simulink model "Prototype"  (R2015a)
settings: Solver=ode45  StartTime=0.0  StopTime=10.0  RelTol=1e-3
undefined symbols (not defined in the file): gray, jet, Rec, SDTV, strel
libraries: visionmorphops x2, visionsinks x2, visionconversions x1, visionanalysis x1, dspvision x1, visiontransforms x1
settings Model: Creator=Andrew H  LastModifiedBy=Andrew H

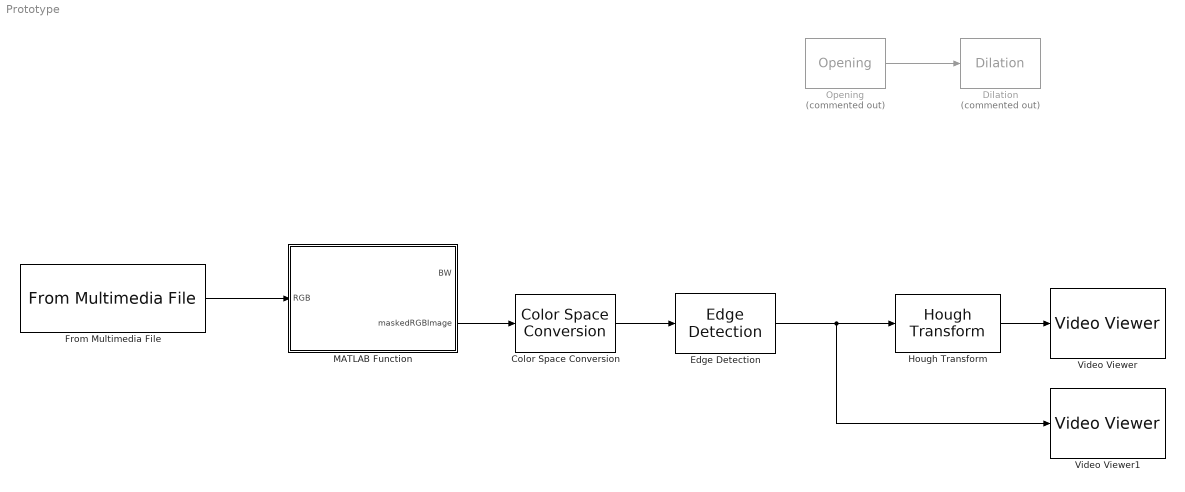
== system Prototype ==
  Color Space Conversion : visionconversions/Color Space  Conversion  conversion=Obsolete  conversionActive=R'G'B' to intensity  wp_str=D65  rec=Rec. 601 (SDTV)  sys=1125/60/2:1  imagePorts=One multidimensional signal
  Dilation : visionmorphops/Dilation  Commented=on  nhoodsrc=Specify via dialog  strel=[1 1; 1 1]
  Edge Detection : visionanalysis/Edge Detection  method=Sobel  outputType=Binary image  userDefinedThreshold=off  thresholdSource=Input port  threshold=20  thresholdTuning=4  edgeThinning=off  threshold_canny=[0.25 0.60]  autoPercent=70  sigma=1  prodOutputMode=Binary point scaling  prodOutputWordLength=32  prodOutputFracLength=8  roundingMode=Floor  overflowMode=off
  From Multimedia File : dspvision/From Multimedia File  inputFilename=C:\Users\Andrew H\Desktop\Video.mp4  loop=on  numPlays=inf  outputStreams=Video only  videoDataType=single  audioDataType=int16  inheritSampleTime=on  userDefinedSampleTime=1/30  noAudioOutput=off  isIntensityVideo=off  fourcc=RGB  colorVideoFormat=One multidimensional signal  outputEOF=off  dataOrg=Column-major  audioFrameSize=1024  computeAudioFrameSize=off  outSamplingMode=Sample based
  Hough Transform : visiontransforms/Hough Transform  theta_res=pi/180  rho_res=1  out_theta_rho=off  outdtmode=double  firstCoeffMode=Binary point scaling  firstCoeffWordLength=16  firstCoeffFracLength=14  secondCoeffMode=Binary point scaling  secondCoeffWordLength=32  secondCoeffFracLength=16  outputMode=Binary point scaling  outputWordLength=16  outputFracLength=0  accumMode=Binary point scaling  accumWordLength=32  accumFracLength=20  prodOutputMode=Binary point scaling  prodOutputWordLength=32  prodOutputFracLength=20  memoryMode=Binary point scaling  memoryWordLength=32  memoryFracLength=16  roundingMode=Nearest  overflowMode=on
  MATLAB Function : MATLAB Function  TreatAsAtomicUnit=on
  Opening : visionmorphops/Opening  Commented=on  nhoodsrc=Specify via dialog  strel=strel('disk', 1)
  Video Viewer : visionsinks/Video Viewer  inputType=Obsolete7b  imagePorts=One multidimensional signal  useColorMap=off  colormapValue=gray(256)  specRange=off  minInputVal=0  maxInputVal=255  FigPos=[970 1021 942 901]  AxisZoom=on  trueSizedOnce=off  OpenAtMdlStart=on  DefaultConfigurationName=vipscopes.VideoViewerScopeCfg
  Video Viewer1 : visionsinks/Video Viewer  inputType=Obsolete7b  imagePorts=One multidimensional signal  useColorMap=off  colormapValue=jet(256)  specRange=off  minInputVal=0  maxInputVal=255  FigPos=[10 1021 942 901]  AxisZoom=on  trueSizedOnce=off  OpenAtMdlStart=on  DefaultConfigurationName=vipscopes.VideoViewerScopeCfg
  wires:
  Opening/1 -> Dilation/1
  Color Space Conversion/1 -> Edge Detection/1
  Edge Detection/1 -> Video Viewer1/1, Hough Transform/1
  Hough Transform/1 -> Video Viewer/1
  From Multimedia File/1 -> MATLAB Function/1(RGB)
  MATLAB Function/2(maskedRGBImage) -> Color Space Conversion/1

== matlab function Prototype/MATLAB Function ==
  data: RGB input; BW output; maskedRGBImage output
function [BW,maskedRGBImage] = createMask(RGB)

% Outputs a BW (binary image) and maskedRGBImage (threshold set using the
% colorThresholder app) from a image/video frame.

%createMask  Threshold RGB image using auto-generated code from colorThresholder app.
%  [BW,MASKEDRGBIMAGE] = createMask(RGB) thresholds image RGB using
%  auto-generated code from the colorThresholder App. The colorspace and
%  minimum/maximum values for each channel of the colorspace were set in the
%  App and result in a binary mask BW and a composite image maskedRGBImage,
%  which shows the original RGB image values under the mask BW.

% Auto-generated by colorThresholder app on 14-Oct-2015
%------------------------------------------------------

% Convert RGB image to chosen color space
I = rgb2hsv(RGB);

% Define thresholds for channel 1 based on histogram settings
channel1Min = 0.952;
channel1Max = 0.094;

% Define thresholds for channel 2 based on histogram settings
channel2Min = 0.025;
channel2Max = 1.000;

% Define thresholds for channel 3 based on histogram settings
channel3Min = 0.724;
channel3Max = 0.967;

% Create mask based on chosen histogram thresholds
BW = ( (I(:,:,1) >= channel1Min) | (I(:,:,1) <= channel1Max) ) & ...
    (I(:,:,2) >= channel2Min ) & (I(:,:,2) <= channel2Max) & ...
    (I(:,:,3) >= channel3Min ) & (I(:,:,3) <= channel3Max);

% Initialize output masked image based on input image.
maskedRGBImage = RGB;

% Set background pixels where BW is false to zero.
maskedRGBImage(repmat(~BW,[1 1 3])) = 0;



% My original Code threshold block
% % Convert RGB image to chosen color space
% I = rgb2hsv(RGB);
% 
% % Define thresholds for channel 1 based on histogram settings
% channel1Min = 0.982;
% channel1Max = 0.235;
% 
% % Define thresholds for channel 2 based on histogram settings
% channel2Min = 0.043;
% channel2Max = 0.655;
% 
% % Define thresholds for channel 3 based on histogram settings
% channel3Min = 0.600;
% channel3Max = 1.000;
% 
% % Create mask based on chosen histogram thresholds
% BW = ( (I(:,:,1) >= channel1Min) | (I(:,:,1) <= channel1Max) ) & ...
%     (I(:,:,2) >= channel2Min ) & (I(:,:,2) <= channel2Max) & ...
%     (I(:,:,3) >= channel3Min ) & (I(:,:,3) <= channel3Max);
% 
% % Initialize output masked image based on input image.
% maskedRGBImage = RGB;
% 
% % Set background pixels where BW is false to zero.
% maskedRGBImage(repmat(~BW,[1 1 3])) = 0;
